simulink subsystem "APPM"  (R2022b)
settings: Solver=VariableStepAuto  StartTime=0.0  StopTime=10.0  RelTol=1e-3
undefined symbols (not defined in the file or in its folder): APP_enuMode
settings Model: DefaultTestHarness=APPS_Harness1  Creator=MAAM  LastModifiedBy=MAAM

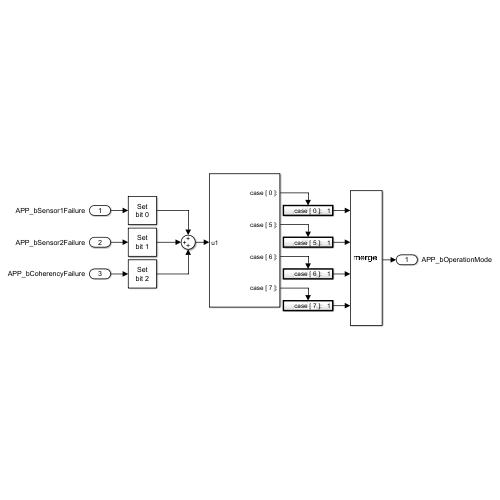
[thumbnail: Simulink's stored preview of the top-level diagram]
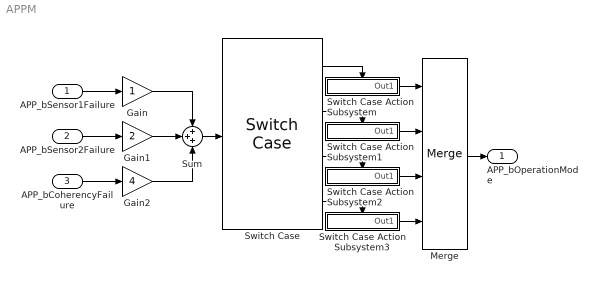
== system APPM ==
  APP_bSensor1Failure : Inport  OutDataTypeStr=boolean
  APP_bSensor2Failure : Inport  Port=2  OutDataTypeStr=boolean
  APP_bCoherencyFailure : Inport  Port=3  OutDataTypeStr=boolean
  Gain : Gain
  Gain1 : Gain  Gain=2
  Gain2 : Gain  Gain=4
  Merge : Merge  Inputs=4
  Sum : Sum  Inputs=+++
  Switch Case : SwitchCase  CaseConditions={0b000, 0b101, 0b110}
  Switch Case Action Subsystem : Subsystem  TreatAsAtomicUnit=on
  Switch Case Action Subsystem1 : Subsystem  TreatAsAtomicUnit=on
  Switch Case Action Subsystem2 : Subsystem  TreatAsAtomicUnit=on
  Switch Case Action Subsystem3 : Subsystem  TreatAsAtomicUnit=on
  APP_bOperationMode : Outport  OutDataTypeStr=Enum: APP_enuMode
  wires:
  Merge/1 -> APP_bOperationMode/1
  Switch Case Action Subsystem3/1(Out1) -> Merge/4
  Switch Case Action Subsystem2/1(Out1) -> Merge/3
  Switch Case Action Subsystem1/1(Out1) -> Merge/2
  Switch Case Action Subsystem/1(Out1) -> Merge/1
  Switch Case/2 -> Switch Case Action Subsystem1/Action
  Switch Case/3 -> Switch Case Action Subsystem2/Action
  Switch Case/4 -> Switch Case Action Subsystem3/Action
  Switch Case/1 -> Switch Case Action Subsystem/Action
  Sum/1 -> Switch Case/1
  Gain2/1 -> Sum/3
  Gain1/1 -> Sum/2
  APP_bSensor1Failure/1 -> Gain/1
  APP_bSensor2Failure/1 -> Gain1/1
  APP_bCoherencyFailure/1 -> Gain2/1
  Gain/1 -> Sum/1

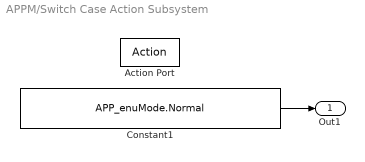
== system APPM/Switch Case Action Subsystem ==
  Action Port : ActionPort
  Constant1 : Constant  Value=APP_enuMode.Normal  OutDataTypeStr=Enum: APP_enuMode
  Out1 : Outport
  wires:
  Constant1/1 -> Out1/1

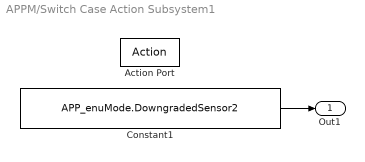
== system APPM/Switch Case Action Subsystem1 ==
  Action Port : ActionPort
  Constant1 : Constant  Value=APP_enuMode.DowngradedSensor2  OutDataTypeStr=Enum: APP_enuMode
  Out1 : Outport
  wires:
  Constant1/1 -> Out1/1

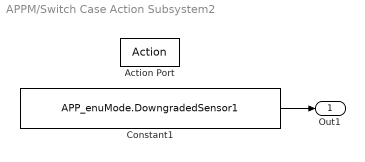
== system APPM/Switch Case Action Subsystem2 ==
  Action Port : ActionPort
  Constant1 : Constant  Value=APP_enuMode.DowngradedSensor1  OutDataTypeStr=Enum: APP_enuMode
  Out1 : Outport
  wires:
  Constant1/1 -> Out1/1

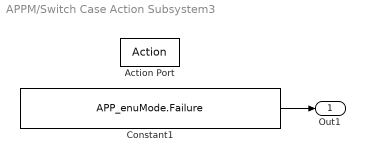
== system APPM/Switch Case Action Subsystem3 ==
  Action Port : ActionPort
  Constant1 : Constant  Value=APP_enuMode.Failure  OutDataTypeStr=Enum: APP_enuMode
  Out1 : Outport
  wires:
  Constant1/1 -> Out1/1
